simulink model "jun23"  (R2018b)
settings: Solver=FixedStepDiscrete  StartTime=0.0  StopTime=7  FixedStep=0.01  RelTol=1e-3
undefined symbols (not defined in the file or in its folder): motorIp, motorSp, Pulsos_vuelta, wheelL, wheelR
libraries: mobileRoboticsTrainingLib x5, simulink x1
settings Model: Creator=Juan David Gómez  LastModifiedBy=Juan David Gómez

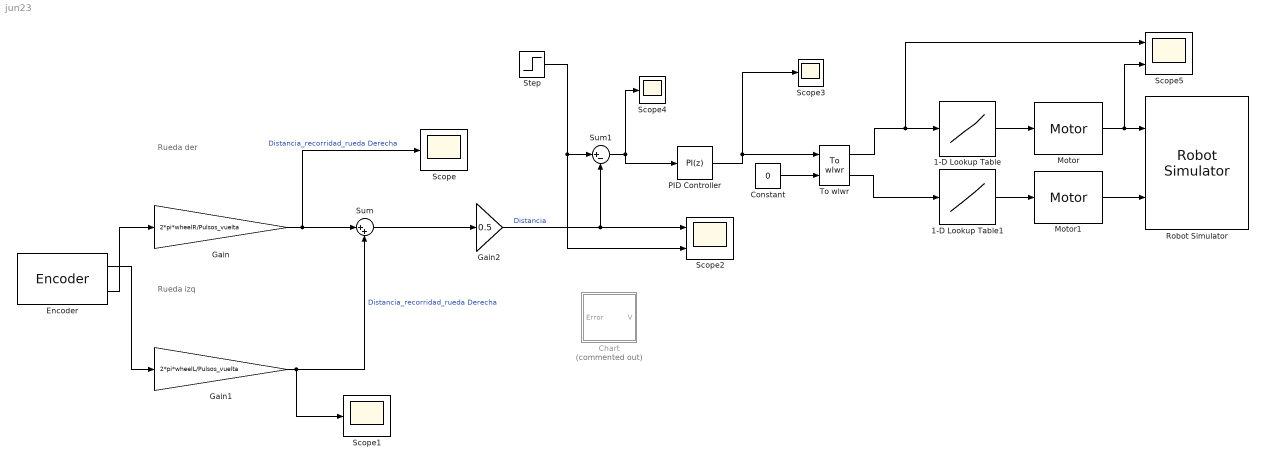
== system jun23 ==
  note: Rueda der
  note: Rueda izq
  1-D Lookup Table : Lookup_n-D  NumberOfTableDimensions=1  BreakpointsForDimension1=motorSp  Table=motorIp  InternalRulePriority=Speed  RndMeth=Simplest  InputSameDT=on
  1-D Lookup Table1 : Lookup_n-D  NumberOfTableDimensions=1  BreakpointsForDimension1=motorSp  Table=motorIp  InternalRulePriority=Speed  RndMeth=Simplest  InputSameDT=on
  Chart : Stateflow chart  Commented=on  TreatAsAtomicUnit=on
  Constant : Constant  Value=0
  Encoder : mobileRoboticsTrainingLib/Encoder  axleLength=L  wheelR=wheelR  ticksPerRot=Pulsos_vuelta
      settings: SourceProductName=Mobile Robotics Training Library
  Gain : Gain  Gain=2*pi*wheelR/Pulsos_vuelta
  Gain1 : Gain  Gain=2*pi*wheelL/Pulsos_vuelta
  Gain2 : Gain  Gain=0.5
  Motor : mobileRoboticsTrainingLib/Motor  motorPlant=wheelMotorModel  sensorType=Speed
      settings: SourceProductName=Mobile Robotics Training Library
  Motor1 : mobileRoboticsTrainingLib/Motor  motorPlant=wheelMotorModel  sensorType=Speed
      settings: SourceProductName=Mobile Robotics Training Library
  PID Controller : simulink/Continuous/PID Controller  Controller=PI  Form=Parallel  TimeDomain=Discrete-time  SampleTime=-1  IntegratorMethod=Forward Euler  FilterMethod=Forward Euler  ControllerParametersSource=internal  P=5  I=3  D=0.1  UseFilter=on  N=100  TunerSelectOption=Transfer Function Based (PID Tuner App)  InitialConditionSource=internal  InitialConditionForIntegrator=0  InitialConditionForFilter=0  DifferentiatorICPrevScaledInput=0  ExternalReset=none  TrackingMode=off  Kt=1  LimitOutput=on  UpperSaturationLimit=0.676  LowerSaturationLimit=-0.676  LinearizeAsGain=on  AntiWindupMode=clamping  Kb=1  POutMin=[]  POutMax=[]  IOutMin=[]  IOutMax=[]  DOutMin=[]  DOutMax=[]  NOutMin=[]  NOutMax=[]  SumOutMin=[]  SumOutMax=[]  SaturationOutMin=[]  SaturationOutMax=[]  PParamMin=[]  PParamMax=[]  IParamMin=[]  IParamMax=[]  DParamMin=[]  DParamMax=[]  NParamMin=[]  NParamMax=[]  KbParamMin=[]  KbParamMax=[]  KtParamMin=[]  KtParamMax=[]  KbOutMin=[]  KbOutMax=[]  KtOutMin=[]  KtOutMax=[]  IntegratorOutMin=[]  IntegratorOutMax=[]  FilterOutMin=[]  FilterOutMax=[]  SumI1OutMin=[]  SumI1OutMax=[]  SumI2OutMin=[]  SumI2OutMax=[]  SumI3OutMin=[]  SumI3OutMax=[]  SumI4OutMin=[]  SumI4OutMax=[]  SumDOutMin=[]  SumDOutMax=[]  DifferentiatorOutMin=[]  DifferentiatorOutMax=[]  FilterDiffOutCoefMin=[]  FilterDiffOutCoefMax=[]  ReciprocalOutMin=[]  ReciprocalOutMax=[]  SumDenOutMin=[]  SumDenOutMax=[]  SumNumOutMin=[]  SumNumOutMax=[]  DivideOutMin=[]  DivideOutMax=[]  IntegratorContinuousStateAttributes=''  IntegratorStateMustResolveToSignalObject=off  IntegratorRTWStateStorageClass=Auto  FilterContinuousStateAttributes=''  FilterStateMustResolveToSignalObject=off  FilterRTWStateStorageClass=Auto  ParallelPVariant=InternalParameters  IdealPVariant=Disabled  IVariant=InternalParameters  DVariant=Disabled  IntegratorVariant=Discrete  SatVariant=Enabled  AWVariant=DiscClampingParallel  PCopyVariant=Disabled  TRVariant=Disabled  FdbkBlocksVariant=Forward  IdealPFdbkVariant=Disabled  SatFdbkVariant=Disabled  DerivativeFilterVariant=Disabled  NVariant=Disabled  NCopyVariant=Disabled_SignalSpec  FilterICVariant=Disabled  IntegratorICVariant=InternalICs  ExternalResetVariant=Disabled  TRSumVariant=Passthrough  SumFdbkVariant=Disabled  SumVariant=Sum_PI  InitialConditionSetting=Output
  Robot Simulator : mobileRoboticsTrainingLib/Robot Simulator  Priority=99  mapVar=[]  startX=1.4461  startY=1.7551  startTheta=0  axleLength=0.15  wheelR=0.03
  Scope{,1,3..4} (4 alike) : Scope
  Scope2 : Scope  NumInputPorts=2
  Scope5 : Scope  NumInputPorts=2
  Step : Step  Time=0  SampleTime=0
  Sum : Sum  Inputs=|++
  Sum1 : Sum  Inputs=|+-
  To wlwr : mobileRoboticsTrainingLib/To wlwr  axleLength=0.15  wheelR=0.03
  wires:
  Encoder/2 -> Gain/1
  Gain/1 -> Sum/1, Scope/1  "Distancia_recorridad_rueda Derecha"
  Gain1/1 -> Sum/2, Scope1/1  "Distancia_recorridad_rueda Derecha"
  Sum/1 -> Gain2/1
  Gain2/1 -> Sum1/2, Scope2/1  "Distancia"
  Encoder/1 -> Gain1/1
  PID Controller/1 -> To wlwr/1, Scope3/1
  Constant/1 -> To wlwr/2
  Step/1 -> Scope2/2, Sum1/1
  Motor1/1 -> Robot Simulator/2
  1-D Lookup Table/1 -> Motor/1
  To wlwr/1 -> Scope5/1, 1-D Lookup Table/1
  1-D Lookup Table1/1 -> Motor1/1
  To wlwr/2 -> 1-D Lookup Table1/1
  Sum1/1 -> PID Controller/1, Scope4/1
  Motor/1 -> Scope5/2, Robot Simulator/1

== stateflow chart jun23/Chart ==
  state Avanza
    V = 0.1
  state Para
    V = 0
  (default) -> Avanza
  Avanza -> Para : [Error <=0]
  data: V output; Error input
